simulink model "DDController"  (R2020a)
settings: Solver=FixedStepAuto  StartTime=0.0  StopTime=10.0  RelTol=1e-3
settings Model: DataDictionary=PCS_Simulation_EnviromentDD.sldd  Creator=ykamatan  LastModifiedBy=ykamatan
settings OptimizationCC: DefaultParameterBehavior=Inlined  EnhancedBackFolding=on  PassReuseOutputArgsAs=Individual arguments  ZeroExternalMemoryAtStartup=off  ZeroInternalMemoryAtStartup=off  OptimizeBlockOrder=speed  DifferentSizesBufferReuse=on  OptimizationCustomize=off  EfficientTunableParamExpr=on
settings DebuggingCC: ParameterTunabilityLossMsg=error
settings ModelReferenceCC: ModelReferenceNumInstancesAllowed=Single
settings SFSimCC: MATLABDynamicMemAlloc=off
settings RTWCC: SystemTargetFile=ert.tlc  TemplateMakefile=ert_default_tmf
settings CodeAppCC: ForceParamTrailComments=on  IgnoreCustomStorageClasses=off  OperatorAnnotations=on  SimulinkDataObjDesc=on  SFDataObjDesc=on  InsertBlockDesc=on
settings ERTTargetCC: TargetLangStandard=C99 (ISO)  GenerateSampleERTMain=on  InlinedParameterPlacement=NonHierarchical  ERTCustomFileTemplate=example_file_process.tlc

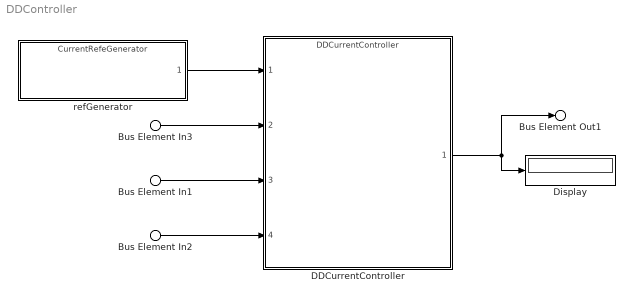
== system DDController ==
  Bus Element In2 : Inport  PortName=SignalsD  Element=Vout
  Bus Element In3 : Inport  PortName=SignalsD  Element=IL
  Bus Element In1 : Inport  PortName=SignalsD  Element=Vin
  DDCurrentController : ModelReference  ModelNameDialog=DDCurrentController.slx  SimulationMode=Normal  ModelReferenceVersion=1.24
  Display : Display
  refGenerator : ModelReference  ModelNameDialog=CurrentRefeGenerator.slx  SimulationMode=Normal  ModelReferenceVersion=1.7
  Bus Element Out1 : Outport  PortName=Duty
  wires:
  DDCurrentController/1 -> Display/1, Bus Element Out1/1
  Bus Element In3/1 -> DDCurrentController/2
  Bus Element In1/1 -> DDCurrentController/3
  Bus Element In2/1 -> DDCurrentController/4
  refGenerator/1 -> DDCurrentController/1
